simulink model "foc_model"  (R2021a)
settings: Solver=VariableStepAuto  StartTime=0.0  StopTime=10.0  RelTol=1e-3
values from neighbouring files (symbols this model uses):
  Gain_I = 26    [foc_model_Initialization.m]
  Gain_P = 7    [foc_model_Initialization.m]
  Id_reference = -50    [foc_model_Initialization.m]
  Iq_reference = 100    [foc_model_Initialization.m]
  Lambda_m = 0.2205    [foc_model_Initialization.m]
  Ld = 1.7e-3    (= 0.0017)    [foc_model_Initialization.m]
  Lq = 3.2e-3    (= 0.0032)    [foc_model_Initialization.m]
  Polepairs = 4    [foc_model_Initialization.m]
  Rs = 0.02    [foc_model_Initialization.m]
libraries: spsControlledVoltageSourceLib x3, spsVoltageMeasurementLib x3, pid_lib x2, spsPermanentMagnetSynchronousMachineLib x1, spsGroundLib x1, eePwmGenerator x1, spspowerguiLib x1
settings Model: Creator=Hidayet  LastModifiedBy=Hidayet

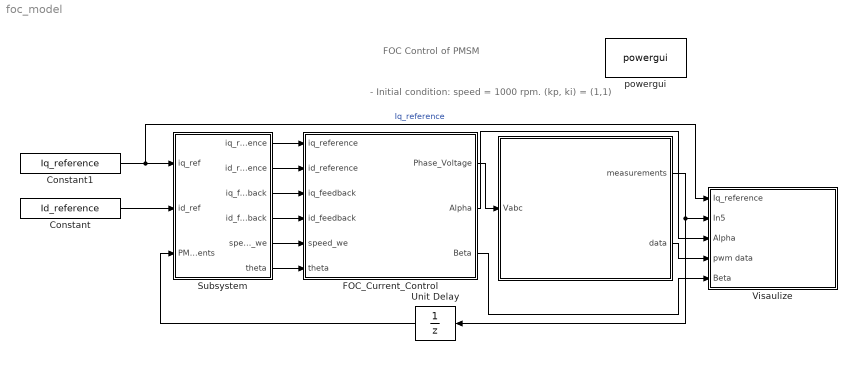
== system foc_model ==
  note: - Initial condition: speed = 1000 rpm. (kp, ki) = (1,1)
  note: FOC Control of PMSM
  " " : Subsystem
  Constant : Constant  Value=Id_reference
  Constant1 : Constant  Value=Iq_reference  VectorParams1D=off
  FOC_Current_Control : Subsystem
  Subsystem : Subsystem
  Unit Delay : UnitDelay  SampleTime=1e-4  HasFrameUpgradeWarning=on
  Visaulize : Subsystem
  powergui : spspowerguiLib/powergui  Priority=1  SimulationMode=Continuous  SampleTime=50e-6  frequency=60  Iterations=50  frequencyindice=0  Pbase=100e6  ErrMax=1e-4  UnitsV=kV  UnitsW=MW  buscounter=0  FunctionMessages=off  echomessages=off  EnableUseOfTLC=off  CurrentSourceSwitches=off  DisableSnubberDevices=off  DisableRonSwitches=off  DisableVfSwitches=off  DisplayEquations=off  AutomaticDiscreteSolvers=off  SolverType=Tustin/Backward Euler (TBE)  Interpol=off  ExternalGateDelay=off  methode=off  Ts=100  x0status=blocks  SPID=on  SwTol=0  HookPort=off  NonlinearTolerance=1e-4  nMaxIteration=100  ContinueOnMaxIteration=off  RestoreLinks=warning  ResistiveCurrentMeasurement=off  Frange=[0:2:500]  Ylog=off  Xlog=on  ShowGrid=off  save=off  variable=ZData  structure=0  ZoomFFT=off  StartTime=0.0  cycles=1  DisplayStyle=1  fundamental=60  FreqAxis=off  MaxFrequency=1000  frequencyindicesteady=1  RmsSteady=1  display=off
  wires:
  Constant1/1 -> Visaulize/1(Iq_reference), Subsystem/1(iq_ref)  "Iq_reference"
  Constant/1 -> Subsystem/2(id_ref)
  Subsystem/1(iq_reference) -> FOC_Current_Control/1(iq_reference)
  Subsystem/2(id_reference) -> FOC_Current_Control/2(id_reference)
  Subsystem/3(iq_feedback) -> FOC_Current_Control/3(iq_feedback)
  Subsystem/4(id_feedback) -> FOC_Current_Control/4(id_feedback)
  Subsystem/5(speed_we) -> FOC_Current_Control/5(speed_we)
  Subsystem/6(theta) -> FOC_Current_Control/6(theta)
  FOC_Current_Control/1(Phase_Voltage) -> " "/1(Vabc)
  " "/1(measurements) -> Unit Delay/1, Visaulize/2(In5)
  Unit Delay/1 -> Subsystem/3(PMSM_Measurements)
  FOC_Current_Control/3(Beta) -> Visaulize/5(Beta)
  FOC_Current_Control/2(Alpha) -> Visaulize/3(Alpha)
  " "/2(data) -> Visaulize/4(pwm data)

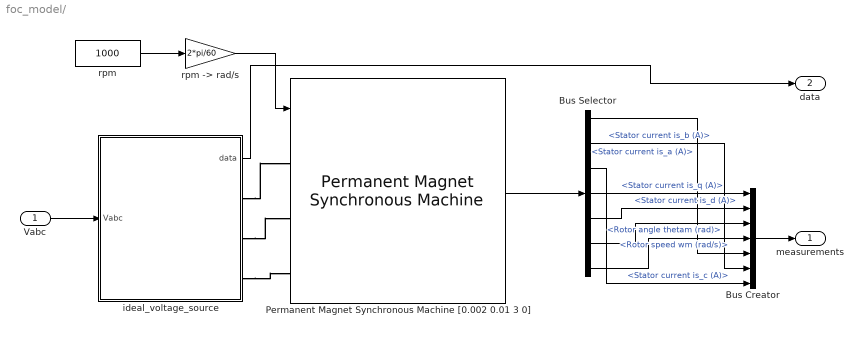
== system foc_model/  ==
  Vabc : Inport
  Bus Creator : BusCreator  Inputs=7
  Bus Selector : BusSelector  OutputSignals=Stator current is_a (A),Stator current is_b (A),Stator current is_c (A),Stator current is_q (A),Stator current is_d (A),Rotor angle thetam (rad),Rotor speed wm (rad/s)
  Permanent Magnet Synchronous Machine [0.002 0.01 3 0] : spsPermanentMagnetSynchronousMachineLib/Permanent Magnet Synchronous Machine  NbPhases=3  FluxDistribution=Sinusoidal  RotorType=Round  MechanicalLoad=Speed w  PresetModel=No  ShowDetailedParameters=on  MeasurementBus=off  Resistance=Rs  Inductance=8.5e-3  dqInductances=[Ld,Lq]  La=La  MachineConstant=Torque Constant (N.m / A_peak)  Flux=0.0014  VoltageCst=1.7775  TorqueCst=0.0147  Flat=120  Mechanical=[0.0027 0.001 4 0]  PolePairs=Polepairs  InitialConditions=[0,0, 0,0]  InitialConditions5ph=[0 0 0 0 0 0]  RefAngle=Aligned with phase A axis (original Park)  IterativeDiscreteModel=Trapezoidal non iterative  TsBlock=-1  TsPowergui=0
  ideal_voltage_source : Subsystem  VariantControl=variantPwm == enumPwm.behavior
  rpm : Constant  Value=1000
  "rpm -> rad/s" : Gain  Gain=2*pi/60
  measurements : Outport  VectorParamsAs1DForOutWhenUnconnected=off
  data : Outport  Port=2
  wires:
  Vabc/1 -> ideal_voltage_source/1(Vabc)
  rpm/1 -> "rpm -> rad/s"/1
  Bus Selector/4 -> Bus Creator/1  "<Stator current is_q (A)>"
  Bus Selector/5 -> Bus Creator/2  "<Stator current is_d (A)>"
  Bus Selector/6 -> Bus Creator/3  "<Rotor angle thetam (rad)>"
  Bus Creator/1 -> measurements/1
  Bus Selector/1 -> Bus Creator/5  "<Stator current is_a (A)>"
  Bus Selector/2 -> Bus Creator/6  "<Stator current is_b (A)>"
  Permanent Magnet Synchronous Machine [0.002 0.01 3 0]/1 -> Bus Selector/1
  Bus Selector/7 -> Bus Creator/4  "<Rotor speed wm (rad/s)>"
  "rpm -> rad/s"/1 -> Permanent Magnet Synchronous Machine [0.002 0.01 3 0]/1
  Bus Selector/3 -> Bus Creator/7  "<Stator current is_c (A)>"
  ideal_voltage_source/1(data) -> data/1
  connections:
  ideal_voltage_source/RConn1 -- Permanent Magnet Synchronous Machine [0.002 0.01 3 0]/LConn1
  ideal_voltage_source/RConn2 -- Permanent Magnet Synchronous Machine [0.002 0.01 3 0]/LConn2
  ideal_voltage_source/RConn3 -- Permanent Magnet Synchronous Machine [0.002 0.01 3 0]/LConn3

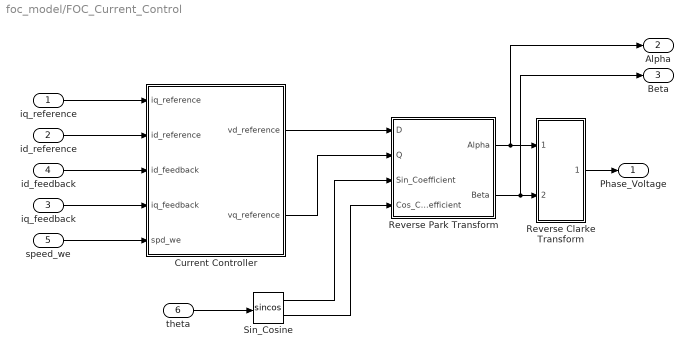
== system foc_model/FOC_Current_Control ==
  iq_reference : Inport  SampleTime=1e-4
  id_reference : Inport  Port=2  SampleTime=1e-4
  iq_feedback : Inport  Port=3  SampleTime=1e-4
  id_feedback : Inport  Port=4  SampleTime=1e-4
  speed_we : Inport  Port=5  SampleTime=1e-4
  theta : Inport  Port=6  SampleTime=1e-4
  Current Controller : Subsystem
  Reverse Clarke Transform : Subsystem
  Reverse Park Transform : Subsystem
  Sin_Cosine : Trigonometry  Operator=sincos
  Phase_Voltage : Outport  SampleTime=1e-4  VectorParamsAs1DForOutWhenUnconnected=off
  Alpha : Outport  Port=2
  Beta : Outport  Port=3
  wires:
  Reverse Clarke Transform/1(ABC) -> Phase_Voltage/1
  Sin_Cosine/2 -> Reverse Park Transform/4(Cos_Coefficient)
  Sin_Cosine/1 -> Reverse Park Transform/3(Sin_Coefficient)
  theta/1 -> Sin_Cosine/1
  Current Controller/2(vq_reference) -> Reverse Park Transform/2(Q)
  Current Controller/1(vd_reference) -> Reverse Park Transform/1(D)
  Reverse Park Transform/1(Alpha) -> Alpha/1, Reverse Clarke Transform/1(Alpha)
  Reverse Park Transform/2(Beta) -> Beta/1, Reverse Clarke Transform/2(Beta)
  id_feedback/1 -> Current Controller/3(id_feedback)
  iq_feedback/1 -> Current Controller/4(iq_feedback)
  speed_we/1 -> Current Controller/5(spd_we)
  iq_reference/1 -> Current Controller/1(iq_reference)
  id_reference/1 -> Current Controller/2(id_reference)

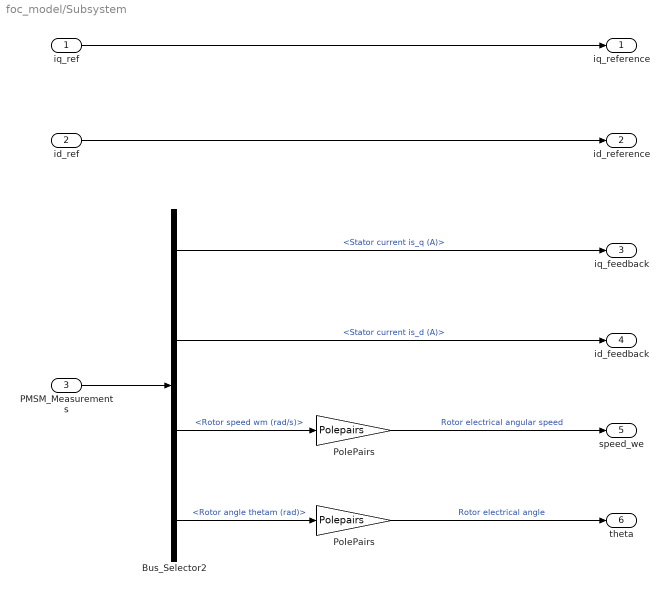
== system foc_model/Subsystem ==
  iq_ref : Inport
  id_ref : Inport  Port=2
  PMSM_Measurements : Inport  Port=3
  Bus_Selector2 : BusSelector  OutputSignals=Stator current is_q (A),Stator current is_d (A),Rotor speed wm (rad/s),Rotor angle thetam (rad)
  PolePairs : Gain  Gain=Polepairs
  "PolePairs " : Gain  Gain=Polepairs
  iq_reference : Outport  VectorParamsAs1DForOutWhenUnconnected=off
  id_reference : Outport  Port=2  VectorParamsAs1DForOutWhenUnconnected=off
  iq_feedback : Outport  Port=3  VectorParamsAs1DForOutWhenUnconnected=off
  id_feedback : Outport  Port=4  VectorParamsAs1DForOutWhenUnconnected=off
  speed_we : Outport  Port=5  VectorParamsAs1DForOutWhenUnconnected=off
  theta : Outport  Port=6  VectorParamsAs1DForOutWhenUnconnected=off
  wires:
  PMSM_Measurements/1 -> Bus_Selector2/1
  PolePairs/1 -> theta/1  "Rotor electrical angle"
  Bus_Selector2/3 -> "PolePairs "/1  "<Rotor speed wm (rad/s)>"
  id_ref/1 -> id_reference/1
  Bus_Selector2/4 -> PolePairs/1  "<Rotor angle thetam (rad)>"
  iq_ref/1 -> iq_reference/1
  Bus_Selector2/2 -> id_feedback/1  "<Stator current is_d (A)>"
  "PolePairs "/1 -> speed_we/1  "Rotor electrical angular speed"
  Bus_Selector2/1 -> iq_feedback/1  "<Stator current is_q (A)>"

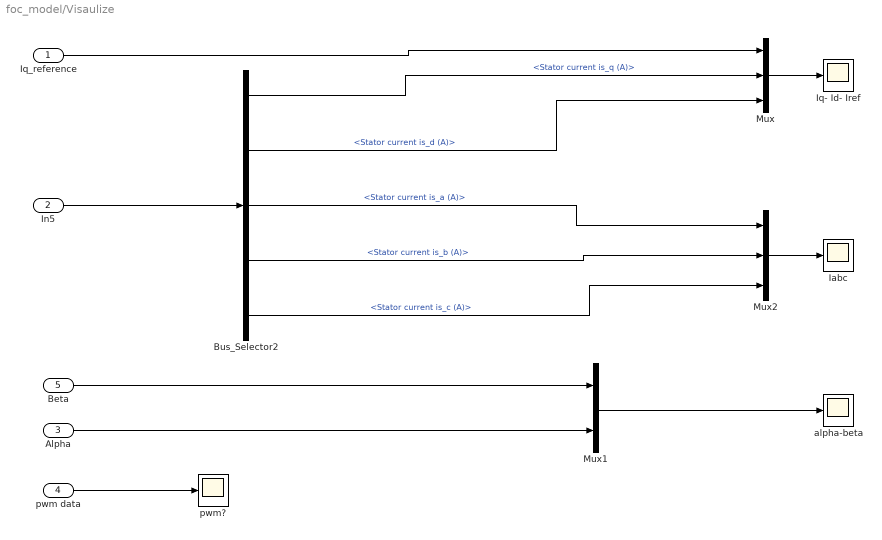
== system foc_model/Visaulize ==
  Iq_reference : Inport
  In5 : Inport  Port=2
  Alpha : Inport  Port=3
  pwm data : Inport  Port=4
  Beta : Inport  Port=5
  Bus_Selector2 : BusSelector  OutputSignals=Stator current is_q (A),Stator current is_d (A),Stator current is_a (A),Stator current is_b (A),Stator current is_c (A)
  Iabc : Scope
  Iq- Id- Iref : Scope
  Mux : Mux  Inputs=3
  Mux1 : Mux  Inputs=2
  Mux2 : Mux  Inputs=3
  alpha-beta : Scope
  pwm? : Scope
  wires:
  In5/1 -> Bus_Selector2/1
  Bus_Selector2/4 -> Mux2/2  "<Stator current is_b (A)>"
  Mux/1 -> Iq- Id- Iref/1
  Bus_Selector2/3 -> Mux2/1  "<Stator current is_a (A)>"
  Bus_Selector2/2 -> Mux/3  "<Stator current is_d (A)>"
  Bus_Selector2/5 -> Mux2/3  "<Stator current is_c (A)>"
  Iq_reference/1 -> Mux/1
  Bus_Selector2/1 -> Mux/2  "<Stator current is_q (A)>"
  Mux2/1 -> Iabc/1
  Beta/1 -> Mux1/1
  Alpha/1 -> Mux1/2
  Mux1/1 -> alpha-beta/1
  pwm data/1 -> pwm?/1

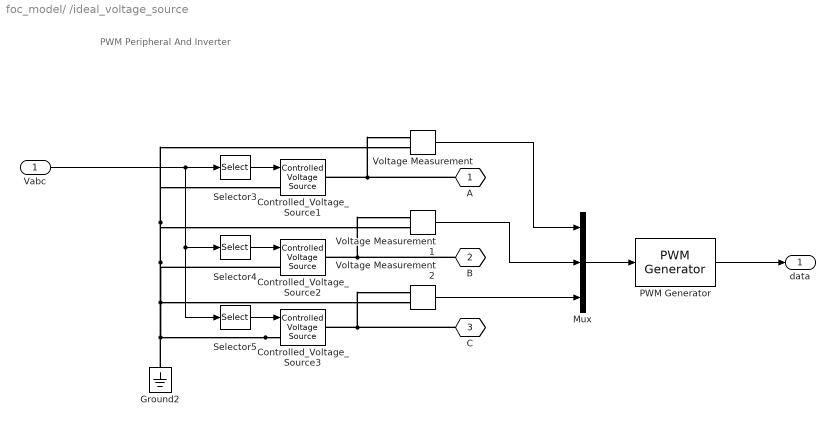
== system foc_model/ /ideal_voltage_source ==
  note: PWM Peripheral And Inverter
  Vabc : Inport
  Controlled_Voltage_Source1 : spsControlledVoltageSourceLib/Controlled Voltage Source  Initialize=off  Source_Type=DC  Amplitude=12  Phase=0  Frequency=0  Measurements=None
  Controlled_Voltage_Source2 : spsControlledVoltageSourceLib/Controlled Voltage Source  Initialize=off  Source_Type=DC  Amplitude=12  Phase=0  Frequency=0  Measurements=None
  Controlled_Voltage_Source3 : spsControlledVoltageSourceLib/Controlled Voltage Source  Initialize=off  Source_Type=DC  Amplitude=12  Phase=0  Frequency=0  Measurements=None
  Ground2 : spsGroundLib/Ground  LConnTagsString=a
  Mux : Mux  Inputs=3
  PWM Generator : eePwmGenerator/PWM Generator  CarrCount=Up  Tper=0.001  Ts=5e-5
  Selector3 : Selector  InputPortWidth=3  IndexOptions=Index vector (dialog)  Indices=[1]  OutputSizes=1
  Selector4 : Selector  InputPortWidth=3  IndexOptions=Index vector (dialog)  Indices=2  OutputSizes=1
  Selector5 : Selector  InputPortWidth=3  IndexOptions=Index vector (dialog)  Indices=3  OutputSizes=1
  Voltage Measurement : spsVoltageMeasurementLib/Voltage Measurement  PhasorSimulation=off  OutputType=Complex  PSBequivalent=0
  Voltage Measurement1 : spsVoltageMeasurementLib/Voltage Measurement  PhasorSimulation=off  OutputType=Complex  PSBequivalent=0
  Voltage Measurement2 : spsVoltageMeasurementLib/Voltage Measurement  PhasorSimulation=off  OutputType=Complex  PSBequivalent=0
  A : PMIOPort  Tag=PMCPort  Side=Right
  B : PMIOPort  Tag=PMCPort  Port=2  Side=Right
  C : PMIOPort  Tag=PMCPort  Port=3  Side=Right
  data : Outport
  wires:
  Vabc/1 -> Selector4/1, Selector5/1, Selector3/1
  Selector5/1 -> Controlled_Voltage_Source3/1
  Selector4/1 -> Controlled_Voltage_Source2/1
  Selector3/1 -> Controlled_Voltage_Source1/1
  Voltage Measurement/1 -> Mux/1
  Voltage Measurement1/1 -> Mux/2
  Voltage Measurement2/1 -> Mux/3
  Mux/1 -> PWM Generator/1
  PWM Generator/1 -> data/1
  connections:
  C/RConn1 -- Voltage Measurement2/LConn1 -- Controlled_Voltage_Source3/RConn1
  B/RConn1 -- Voltage Measurement1/LConn1 -- Controlled_Voltage_Source2/RConn1
  A/RConn1 -- Voltage Measurement/LConn1 -- Controlled_Voltage_Source1/RConn1
  Controlled_Voltage_Source3/LConn1 -- Voltage Measurement1/LConn2 -- Voltage Measurement/LConn2 -- Controlled_Voltage_Source1/LConn1 -- Controlled_Voltage_Source2/LConn1 -- Voltage Measurement2/LConn2 -- Ground2/LConn1

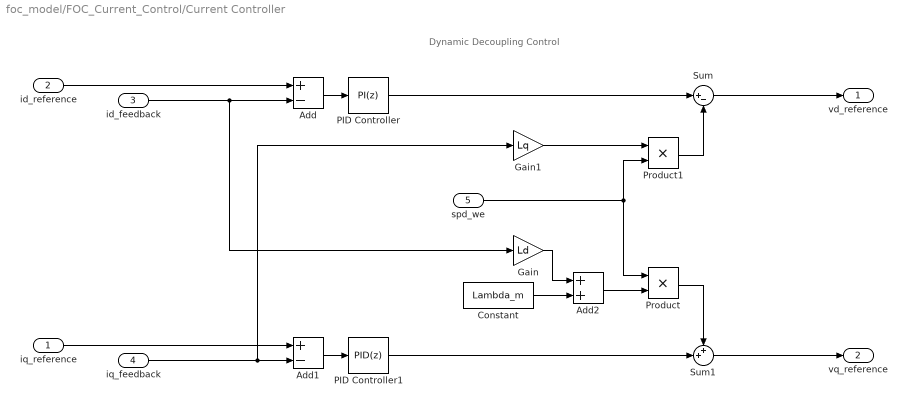
== system foc_model/FOC_Current_Control/Current Controller ==
  note: Dynamic Decoupling Control
  iq_reference : Inport  SampleTime=1e-4
  id_reference : Inport  Port=2  SampleTime=1e-4
  id_feedback : Inport  Port=3  SampleTime=1e-4
  iq_feedback : Inport  Port=4  SampleTime=1e-4
  spd_we : Inport  Port=5  SampleTime=1e-4
  Add : Sum  Inputs=+-
  Add1 : Sum  Inputs=+-
  Add2 : Sum
  Constant : Constant  Value=Lambda_m  SampleTime=1e-4
  Gain : Gain  Gain=Ld
  Gain1 : Gain  Gain=Lq
  PID Controller : pid_lib/PID Controller  Controller=PI  Form=Parallel  TimeDomain=Discrete-time  UseExternalTs=off  SampleTime=-1  IntegratorMethod=Forward Euler  FilterMethod=Forward Euler  ControllerParametersSource=internal  P=Gain_P  I=Gain_I  D=0  UseFilter=on  N=100  TunerSelectOption=Transfer Function Based (PID Tuner App)  InitialConditionSource=internal  InitialConditionForIntegrator=0  InitialConditionForFilter=0  DifferentiatorICPrevScaledInput=0  ExternalReset=none  TrackingMode=off  Kt=1  LimitOutput=off  SatLimitsSource=internal  UpperSaturationLimit=inf  LowerSaturationLimit=-inf  LinearizeAsGain=on  AntiWindupMode=none  Kb=1  POutMin=[]  POutMax=[]  IOutMin=[]  IOutMax=[]  DOutMin=[]  DOutMax=[]  NOutMin=[]  NOutMax=[]  SumOutMin=[]  SumOutMax=[]  SaturationOutMin=[]  SaturationOutMax=[]  PParamMin=[]  PParamMax=[]  IParamMin=[]  IParamMax=[]  DParamMin=[]  DParamMax=[]  NParamMin=[]  NParamMax=[]  KbParamMin=[]  KbParamMax=[]  KtParamMin=[]  KtParamMax=[]  KbOutMin=[]  KbOutMax=[]  KtOutMin=[]  KtOutMax=[]  IntegratorOutMin=[]  IntegratorOutMax=[]  FilterOutMin=[]  FilterOutMax=[]  SumI1OutMin=[]  SumI1OutMax=[]  SumI2OutMin=[]  SumI2OutMax=[]  SumI3OutMin=[]  SumI3OutMax=[]  SumI4OutMin=[]  SumI4OutMax=[]  SumDOutMin=[]  SumDOutMax=[]  DifferentiatorOutMin=[]  DifferentiatorOutMax=[]  FilterDiffOutCoefMin=[]  FilterDiffOutCoefMax=[]  ReciprocalOutMin=[]  ReciprocalOutMax=[]  SumDenOutMin=[]  SumDenOutMax=[]  SumNumOutMin=[]  SumNumOutMax=[]  DivideOutMin=[]  DivideOutMax=[]  UdiffTsProdOutMin=[]  UdiffTsProdOutMax=[]  NTsProdOutMin=[]  NTsProdOutMax=[]  UintegralTsProdOutMin=[]  UintegralTsProdOutMax=[]  UngainTsProdOutMin=[]  UngainTsProdOutMax=[]  IntegratorContinuousStateAttributes=''  IntegratorStateMustResolveToSignalObject=off  IntegratorRTWStateStorageClass=Auto  FilterContinuousStateAttributes=''  FilterStateMustResolveToSignalObject=off  FilterRTWStateStorageClass=Auto  ParallelPVariant=InternalParameters  IdealPVariant=Disabled  IVariant=InternalParameters  DVariant=Disabled  IntegratorVariant=Discrete  SatVariant=Disabled  AWVariant=Passthrough  PCopyVariant=Disabled  TRVariant=Disabled  FdbkBlocksVariant=Forward  IdealPFdbkVariant=Disabled  SatFdbkVariant=Disabled  DerivativeFilterVariant=Disabled  NVariant=Disabled  NCopyVariant=Disabled_SignalSpec  FilterICVariant=Disabled  IntegratorICVariant=InternalICs  ExternalResetVariant=Disabled  TRSumVariant=Passthrough  SumFdbkVariant=Disabled  SumVariant=Sum_PI  TsampFilterVariant=InternalTs  TsampNgainVariant=Passthrough  TsampIntegralVariant=Passthrough  ExternalSaturationOutDataTypeStr=Inherit: Same as second input
  PID Controller1 : pid_lib/PID Controller  Controller=PID  Form=Parallel  TimeDomain=Discrete-time  UseExternalTs=off  SampleTime=-1  IntegratorMethod=Forward Euler  FilterMethod=Forward Euler  ControllerParametersSource=internal  P=Gain_P  I=Gain_I  D=0  UseFilter=on  N=100  TunerSelectOption=Transfer Function Based (PID Tuner App)  InitialConditionSource=internal  InitialConditionForIntegrator=0  InitialConditionForFilter=0  DifferentiatorICPrevScaledInput=0  ExternalReset=none  TrackingMode=off  Kt=1  LimitOutput=off  SatLimitsSource=internal  UpperSaturationLimit=inf  LowerSaturationLimit=-inf  LinearizeAsGain=on  AntiWindupMode=none  Kb=1  POutMin=[]  POutMax=[]  IOutMin=[]  IOutMax=[]  DOutMin=[]  DOutMax=[]  NOutMin=[]  NOutMax=[]  SumOutMin=[]  SumOutMax=[]  SaturationOutMin=[]  SaturationOutMax=[]  PParamMin=[]  PParamMax=[]  IParamMin=[]  IParamMax=[]  DParamMin=[]  DParamMax=[]  NParamMin=[]  NParamMax=[]  KbParamMin=[]  KbParamMax=[]  KtParamMin=[]  KtParamMax=[]  KbOutMin=[]  KbOutMax=[]  KtOutMin=[]  KtOutMax=[]  IntegratorOutMin=[]  IntegratorOutMax=[]  FilterOutMin=[]  FilterOutMax=[]  SumI1OutMin=[]  SumI1OutMax=[]  SumI2OutMin=[]  SumI2OutMax=[]  SumI3OutMin=[]  SumI3OutMax=[]  SumI4OutMin=[]  SumI4OutMax=[]  SumDOutMin=[]  SumDOutMax=[]  DifferentiatorOutMin=[]  DifferentiatorOutMax=[]  FilterDiffOutCoefMin=[]  FilterDiffOutCoefMax=[]  ReciprocalOutMin=[]  ReciprocalOutMax=[]  SumDenOutMin=[]  SumDenOutMax=[]  SumNumOutMin=[]  SumNumOutMax=[]  DivideOutMin=[]  DivideOutMax=[]  UdiffTsProdOutMin=[]  UdiffTsProdOutMax=[]  NTsProdOutMin=[]  NTsProdOutMax=[]  UintegralTsProdOutMin=[]  UintegralTsProdOutMax=[]  UngainTsProdOutMin=[]  UngainTsProdOutMax=[]  IntegratorContinuousStateAttributes=''  IntegratorStateMustResolveToSignalObject=off  IntegratorRTWStateStorageClass=Auto  FilterContinuousStateAttributes=''  FilterStateMustResolveToSignalObject=off  FilterRTWStateStorageClass=Auto  ParallelPVariant=InternalParameters  IdealPVariant=Disabled  IVariant=InternalParameters  DVariant=InternalParameters  IntegratorVariant=Discrete  SatVariant=Disabled  AWVariant=Passthrough  PCopyVariant=Disabled  TRVariant=Disabled  FdbkBlocksVariant=Forward  IdealPFdbkVariant=Disabled  SatFdbkVariant=Disabled  DerivativeFilterVariant=ForwardEulerFilter  NVariant=InternalParameters  NCopyVariant=Disabled  FilterICVariant=InternalICsFilter  IntegratorICVariant=InternalICs  ExternalResetVariant=Disabled  TRSumVariant=Passthrough  SumFdbkVariant=Disabled  SumVariant=Sum_PID  TsampFilterVariant=InternalTs  TsampNgainVariant=Passthrough  TsampIntegralVariant=Passthrough  ExternalSaturationOutDataTypeStr=Inherit: Same as second input
  Product : Product
  Product1 : Product
  Sum : Sum  Inputs=|+-
  Sum1 : Sum  Inputs=++|
  vd_reference : Outport  SampleTime=1e-4  VectorParamsAs1DForOutWhenUnconnected=off
  vq_reference : Outport  Port=2  SampleTime=1e-4  VectorParamsAs1DForOutWhenUnconnected=off
  wires:
  Sum/1 -> vd_reference/1
  PID Controller/1 -> Sum/1
  id_feedback/1 -> Gain/1, Add/2
  Add/1 -> PID Controller/1
  iq_feedback/1 -> Gain1/1, Add1/2
  id_reference/1 -> Add/1
  Add1/1 -> PID Controller1/1
  iq_reference/1 -> Add1/1
  Sum1/1 -> vq_reference/1
  PID Controller1/1 -> Sum1/2
  Gain/1 -> Add2/1
  Constant/1 -> Add2/2
  Add2/1 -> Product/2
  spd_we/1 -> Product1/2, Product/1
  Gain1/1 -> Product1/1
  Product1/1 -> Sum/2
  Product/1 -> Sum1/1

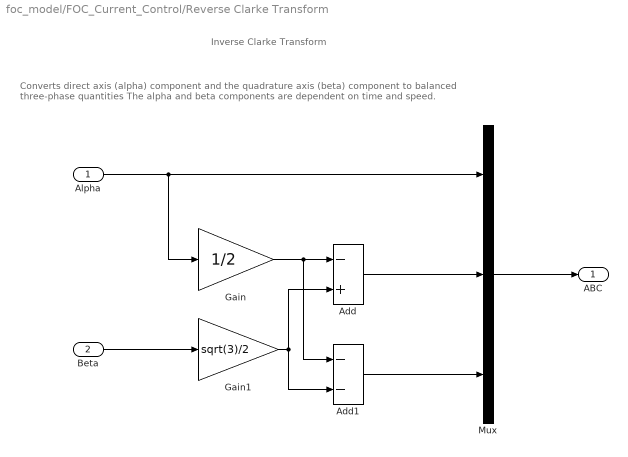
== system foc_model/FOC_Current_Control/Reverse Clarke Transform ==
  note: Inverse Clarke Transform
  note: Converts direct axis (alpha) component and the quadrature axis (beta) component to balanced three-phase quantities
      | The alpha and beta components are dependent on time and speed.
  Alpha : Inport
  Beta : Inport  Port=2
  Add : Sum  Inputs=-+  OutDataTypeStr=Inherit: Same as first input
  Add1 : Sum  Inputs=--  OutDataTypeStr=Inherit: Same as first input
  Gain : Gain  Gain=1/2
  Gain1 : Gain  Gain=sqrt(3)/2
  Mux : Mux  Inputs=3
  ABC : Outport  VectorParamsAs1DForOutWhenUnconnected=off
  wires:
  Beta/1 -> Gain1/1
  Mux/1 -> ABC/1
  Alpha/1 -> Mux/1, Gain/1
  Add1/1 -> Mux/3
  Gain1/1 -> Add1/2, Add/2
  Gain/1 -> Add1/1, Add/1
  Add/1 -> Mux/2

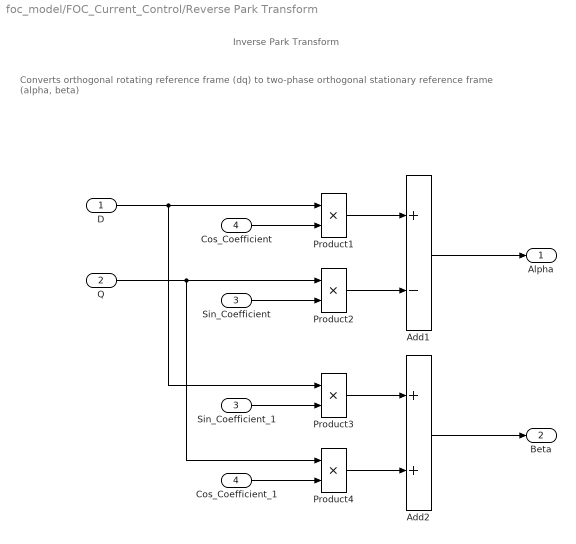
== system foc_model/FOC_Current_Control/Reverse Park Transform ==
  note: Converts orthogonal rotating reference frame (dq) to two-phase orthogonal stationary reference frame (alpha, beta)
  note: Inverse Park Transform
  D : Inport
  Q : Inport  Port=2
  Sin_Coefficient : Inport  Port=3
  Cos_Coefficient : Inport  Port=4
  Add1 : Sum  Inputs=+-  OutDataTypeStr=Inherit: Same as first input
  Add2 : Sum  OutDataTypeStr=Inherit: Same as first input
  Cos_Coefficient_1 : InportShadow  Port=4
  Product{1..4} (4 alike) : Product  RndMeth=Simplest
  Sin_Coefficient_1 : InportShadow  Port=3
  Alpha : Outport  VectorParamsAs1DForOutWhenUnconnected=off
  Beta : Outport  Port=2  VectorParamsAs1DForOutWhenUnconnected=off
  wires:
  Sin_Coefficient_1/1 -> Product3/2
  Product2/1 -> Add1/2
  Cos_Coefficient_1/1 -> Product4/2
  Add2/1 -> Beta/1
  Product3/1 -> Add2/1
  Add1/1 -> Alpha/1
  Product1/1 -> Add1/1
  Product4/1 -> Add2/2
  Sin_Coefficient/1 -> Product2/2
  D/1 -> Product3/1, Product1/1
  Q/1 -> Product2/1, Product4/1
  Cos_Coefficient/1 -> Product1/2
